simulink library "arduinopio_lib"  (R2025b)
settings: Solver=VariableStepAuto  StartTime=0.0  StopTime=10.0  RelTol=1e-3
undefined symbols (not defined in the file): ESP32, WROOM
settings Model: Creator=admin  LastModifiedBy=admin

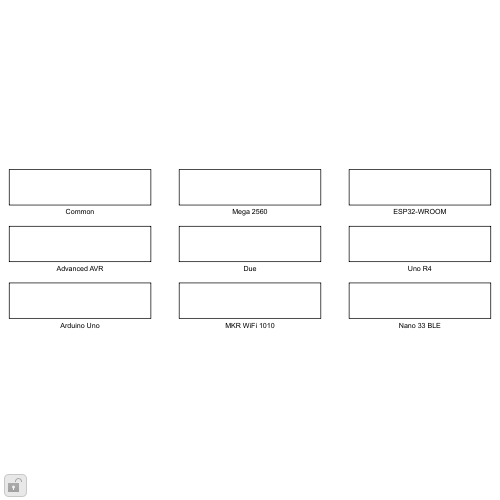
[thumbnail: Simulink's stored preview of the top-level diagram]
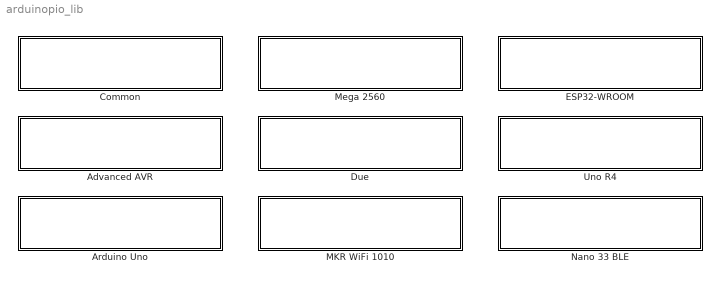
== system arduinopio_lib ==
  Advanced AVR : Subsystem
  Arduino Uno : Subsystem
  Common : Subsystem
  Due : Subsystem
  ESP32-WROOM : Subsystem
  MKR WiFi 1010 : Subsystem
  Mega 2560 : Subsystem
  Nano 33 BLE : Subsystem
  Uno R4 : Subsystem

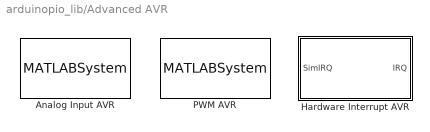
== system arduinopio_lib/Advanced AVR ==
  Analog Input AVR : MATLABSystem  System=arduinopio.blocks.avr.AnalogInputAvr  Pin=0  ReferenceSelect=1  PrescalerSelect=7  SampleTime=-1  SimulateUsing=Code generation
      mask Type: arduinopio.blocks.avr.AnalogInputAvr
  Hardware Interrupt AVR : Subsystem  mask(Arduino PIO Hardware Interrupt AVR){SourceId=0}
      mask prompts: SourceId "SourceId (0=T1 ovf, 1=T1 cmpA, 2=T2 ovf, 3=ADC)"
      mask help: 0=Timer1 overflow, 1=Timer1 compare A, 2=Timer2 overflow, 3=ADC complete.
      mask init:
      | set_param([gcb '/Driver'], 'SourceId', SourceId);
      mask Display: disp('Hardware Interrupt AVR')
  PWM AVR : MATLABSystem  System=arduinopio.blocks.avr.PwmAvr  Pin=5  PrescalerSelect=3  FastPwm=on  SampleTime=-1  SimulateUsing=Code generation
      mask Type: arduinopio.blocks.avr.PwmAvr

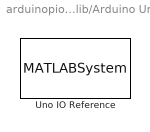
== system arduinopio_lib/Arduino Uno ==
  Uno IO Reference : MATLABSystem  System=arduinopio.blocks.uno.IoReference  SimulateUsing=Code generation
      mask Type: arduinopio.blocks.uno.IoReference

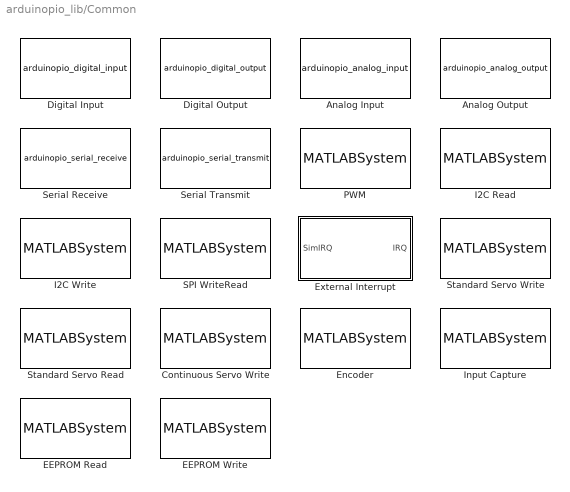
== system arduinopio_lib/Common ==
  Analog Input : M-S-Function  FunctionName=arduinopio_analog_input  Parameters=Pin, SampleTime, SimValue  mask(Arduino PIO Analog Input){Pin=0, SampleTime=-1, SimValue=0}
      mask prompts: Pin "Analog pin (0 = A0)"; SampleTime "Sample time (-1 = inherited)"; SimValue "Simulation ADC counts (0-1023)"
      mask help: Uno A0-A5 as pin 0-5. Output is 0-1023 for a 10-bit ADC.
      mask Display: disp('Analog Input')
  Analog Output : M-S-Function  FunctionName=arduinopio_analog_output  Parameters=Pin, SampleTime  mask(Arduino PIO Analog Output){Pin=5, SampleTime=-1}
      mask prompts: Pin "PWM pin"; SampleTime "Sample time (-1 = inherited)"
      mask help: Arduino analogWrite on a PWM pin. Input is 0-255. Uno PWM pins: 3, 5, 6, 9, 10, 11.
      mask Display: disp('Analog Output')
  Continuous Servo Write : MATLABSystem  System=arduinopio.blocks.common.ContinuousServoWrite  Pin=9  SampleTime=-1  SimulateUsing=Code generation
      mask Type: arduinopio.blocks.common.ContinuousServoWrite
  Digital Input : M-S-Function  FunctionName=arduinopio_digital_input  Parameters=Pin, Pullup, SampleTime, SimValue  mask(Arduino PIO Digital Input){Pin=2, EnablePullup=off, SampleTime=-1, SimValue=0}
      mask prompts: Pin "Pin number"; EnablePullup "Enable pull-up"; SampleTime "Sample time (-1 = inherited)"; SimValue "Simulation output (0 or 1)"
      mask help: Read a digital pin. Uno pins 0-13 and A0-A5 (14-19) are valid.
      mask init:
      | Pullup = double(strcmp(EnablePullup, 'on'));
      mask Display: disp('Digital Input')
  Digital Output : M-S-Function  FunctionName=arduinopio_digital_output  Parameters=Pin, SampleTime  mask(Arduino PIO Digital Output){Pin=13, SampleTime=-1}
      mask prompts: Pin "Pin number"; SampleTime "Sample time (-1 = inherited)"
      mask help: Write a digital pin. Uno LED_BUILTIN is pin 13.
      mask Display: disp('Digital Output')
  EEPROM Read : MATLABSystem  System=arduinopio.blocks.common.EepromRead  StartAddress=0  DataLength=1  SampleTime=-1  SimulateUsing=Code generation
      mask Type: arduinopio.blocks.common.EepromRead
  EEPROM Write : MATLABSystem  System=arduinopio.blocks.common.EepromWrite  StartAddress=0  SampleTime=-1  SimulateUsing=Code generation
      mask Type: arduinopio.blocks.common.EepromWrite
  Encoder : MATLABSystem  System=arduinopio.blocks.common.Encoder  PinA=2  PinB=3  ResetEachSample=off  SampleTime=-1  SimulateUsing=Code generation
      mask Type: arduinopio.blocks.common.Encoder
  External Interrupt : Subsystem  mask(Arduino PIO External Interrupt){Pin=2, Mode=3, EnablePullup=off}
      mask prompts: Pin "Pin number (Uno: 2 or 3)"; Mode "Mode (0=LOW, 1=CHANGE, 2=FALLING, 3=RISING)"; EnablePullup "Enable pull-up"
      mask help: Uno INT0/INT1 (pins 2 and 3). Connect IRQ to a Function-Call Subsystem. SimIRQ is simulation-only.
      mask init:
      | set_param([gcb '/Driver'], 'Pin', Pin);
      | set_param([gcb '/Driver'], 'Mode', Mode);
      | set_param([gcb '/Driver'], 'EnablePullup', EnablePullup);
      mask Display: disp('External Interrupt')
  I2C Read : MATLABSystem  System=arduinopio.blocks.common.I2cRead  SlaveAddress=8  HasRegister=on  RegisterAddress=0  DataLength=1  SampleTime=-1  SimulateUsing=Code generation
      mask Type: arduinopio.blocks.common.I2cRead
  I2C Write : MATLABSystem  System=arduinopio.blocks.common.I2cWrite  SlaveAddress=8  HasRegister=on  RegisterAddress=0  SampleTime=-1  SimulateUsing=Code generation
      mask Type: arduinopio.blocks.common.I2cWrite
  Input Capture : MATLABSystem  System=arduinopio.blocks.common.InputCapture  Pin=8  SampleTime=-1  SimulateUsing=Code generation
      mask Type: arduinopio.blocks.common.InputCapture
  PWM : MATLABSystem  System=arduinopio.blocks.common.Pwm  Pin=5  SampleTime=-1  SimulateUsing=Code generation
      mask Type: arduinopio.blocks.common.Pwm
  SPI WriteRead : MATLABSystem  System=arduinopio.blocks.common.SpiWriteRead  ChipSelectPin=10  ClockHz=4000000  SpiMode=0  MsbFirst=on  SampleTime=-1  SimulateUsing=Code generation
      mask Type: arduinopio.blocks.common.SpiWriteRead
  Serial Receive : M-S-Function  FunctionName=arduinopio_serial_receive  Parameters=Port, BaudRate, DataLength, SampleTime  mask(Arduino PIO Serial Receive){Port=0, BaudRate=9600, DataLength=1, SampleTime=-1}
      mask prompts: Port "UART port index"; BaudRate "Baud rate"; DataLength "Bytes per step"; SampleTime "Sample time (-1 = inherited)"
      mask help: Read bytes from hardware UART. Uno uses Serial0 on pins 0 and 1.
      mask Display: disp('Serial Receive')
  Serial Transmit : M-S-Function  FunctionName=arduinopio_serial_transmit  Parameters=Port, BaudRate, SampleTime  mask(Arduino PIO Serial Transmit){Port=0, BaudRate=9600, SampleTime=-1}
      mask prompts: Port "UART port index"; BaudRate "Baud rate"; SampleTime "Sample time (-1 = inherited)"
      mask help: Write uint8 bytes to hardware UART. Uno uses Serial0 on pins 0 and 1.
      mask Display: disp('Serial Transmit')
  Standard Servo Read : MATLABSystem  System=arduinopio.blocks.common.StandardServoRead  Pin=9  SampleTime=-1  SimulateUsing=Code generation
      mask Type: arduinopio.blocks.common.StandardServoRead
  Standard Servo Write : MATLABSystem  System=arduinopio.blocks.common.StandardServoWrite  Pin=9  SampleTime=-1  SimulateUsing=Code generation
      mask Type: arduinopio.blocks.common.StandardServoWrite

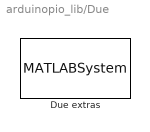
== system arduinopio_lib/Due ==
  Due extras : MATLABSystem  System=arduinopio.blocks.BoardStub  BoardName=Arduino Due  ExtraBlocks=Analog Output (DAC),On-board CAN,Serial1-3  SimulateUsing=Code generation
      mask Type: arduinopio.blocks.BoardStub

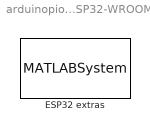
== system arduinopio_lib/ESP32-WROOM ==
  ESP32 extras : MATLABSystem  System=arduinopio.blocks.BoardStub  BoardName=ESP32-WROOM  ExtraBlocks=Analog Output,WiFi TCP/UDP,BLE,Touch Sense  SimulateUsing=Code generation
      mask Type: arduinopio.blocks.BoardStub

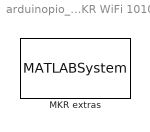
== system arduinopio_lib/MKR WiFi 1010 ==
  MKR extras : MATLABSystem  System=arduinopio.blocks.BoardStub  BoardName=Arduino MKR WiFi 1010  ExtraBlocks=Analog Output,WiFi TCP/UDP,BLE  SimulateUsing=Code generation
      mask Type: arduinopio.blocks.BoardStub

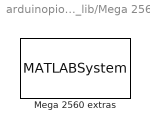
== system arduinopio_lib/Mega 2560 ==
  Mega 2560 extras : MATLABSystem  System=arduinopio.blocks.BoardStub  BoardName=Arduino Mega 2560  ExtraBlocks=Serial1,Serial2,Serial3,More PWM/ADC pins  SimulateUsing=Code generation
      mask Type: arduinopio.blocks.BoardStub

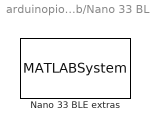
== system arduinopio_lib/Nano 33 BLE ==
  Nano 33 BLE extras : MATLABSystem  System=arduinopio.blocks.BoardStub  BoardName=Arduino Nano 33 BLE Sense  ExtraBlocks=Analog Output,BLE Receive,BLE Transmit  SimulateUsing=Code generation
      mask Type: arduinopio.blocks.BoardStub

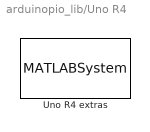
== system arduinopio_lib/Uno R4 ==
  Uno R4 extras : MATLABSystem  System=arduinopio.blocks.BoardStub  BoardName=Arduino Uno R4  ExtraBlocks=Analog Output,On-board CAN,12x8 LED Matrix,WiFi (WiFi model)  SimulateUsing=Code generation
      mask Type: arduinopio.blocks.BoardStub

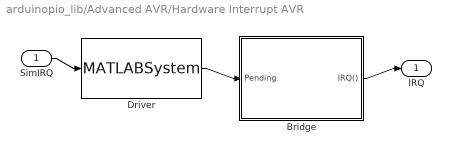
== system arduinopio_lib/Advanced AVR/Hardware Interrupt AVR ==
  SimIRQ : Inport  OutDataTypeStr=boolean
  Bridge : Stateflow chart  TreatAsAtomicUnit=on
  Driver : MATLABSystem  System=arduinopio.blocks.avr.HardwareInterruptAvr  SourceId=0  SampleTime=-1  SimulateUsing=Code generation
      mask Type: arduinopio.blocks.avr.HardwareInterruptAvr
  IRQ : Outport
  wires:
  SimIRQ/1 -> Driver/1
  Driver/1 -> Bridge/1(Pending)
  Bridge/1(IRQ()) -> IRQ/1

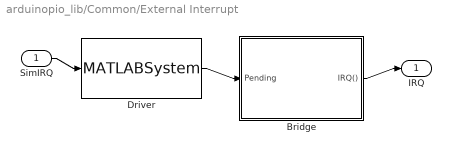
== system arduinopio_lib/Common/External Interrupt ==
  SimIRQ : Inport  OutDataTypeStr=boolean
  Bridge : Stateflow chart  TreatAsAtomicUnit=on
  Driver : MATLABSystem  System=arduinopio.blocks.common.ExternalInterrupt  Pin=2  Mode=3  EnablePullup=off  SampleTime=-1  SimulateUsing=Code generation
      mask Type: arduinopio.blocks.common.ExternalInterrupt
  IRQ : Outport
  wires:
  SimIRQ/1 -> Driver/1
  Driver/1 -> Bridge/1(Pending)
  Bridge/1(IRQ()) -> IRQ/1

== stateflow chart arduinopio_lib/Common/External Interrupt/Bridge ==
  state Poll
    during:
    if Pending
    send(IRQ);
    end
  data: Pending input boolean
  events: IRQ output FUNCTION_CALL_EVENT

== stateflow chart arduinopio_lib/Advanced AVR/Hardware Interrupt AVR/Bridge ==
  state Poll
    during:
    if Pending
    send(IRQ);
    end
  data: Pending input boolean
  events: IRQ output FUNCTION_CALL_EVENT
